simulink model "Single_track_Drift_model"  (R2024b)
settings: Solver=ode45  StartTime=0.0  StopTime=10.0  RelTol=1e-3
settings Model: Creator=fanny  LastModifiedBy=fanny

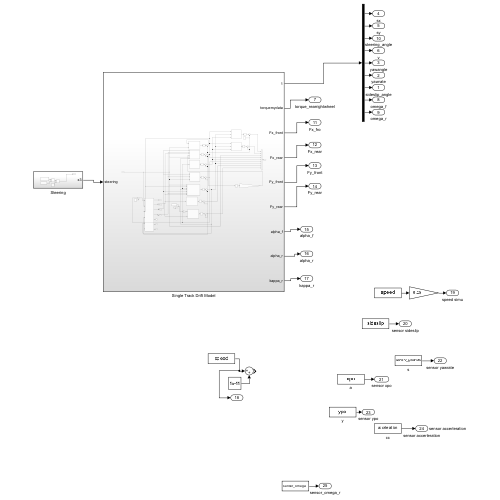
[thumbnail: Simulink's stored preview of the top-level diagram]
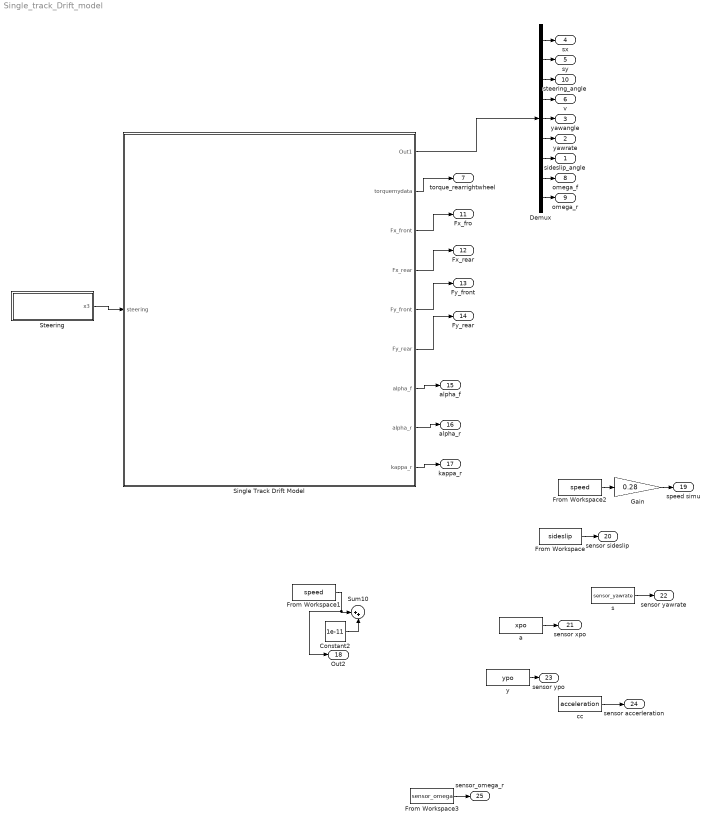
== system Single_track_Drift_model ==
  Constant2 : Constant  Value=1e-11
  Demux : Demux  Outputs=9
  From Workspace : FromWorkspace  VariableName=sideslip
  From Workspace1 : FromWorkspace  VariableName=speed
  From Workspace2 : FromWorkspace  VariableName=speed
  From Workspace3 : FromWorkspace  VariableName=sensor_omega
  Gain : Gain  Gain=0.28
  Single Track Drift Model : Subsystem
  Steering : Subsystem
  Sum10 : Sum  Inputs=|++
  a : FromWorkspace  VariableName=xpo
  cc : FromWorkspace  VariableName=acceleration
  s : FromWorkspace  VariableName=sensor_yawrate
  y : FromWorkspace  VariableName=ypo
  sideslip_angle : Outport
  yawrate : Outport  Port=2
  yawangle : Outport  Port=3
  sx : Outport  Port=4
  sy : Outport  Port=5
  v : Outport  Port=6
  torque_rearrightwheel : Outport  Port=7
  omega_f : Outport  Port=8
  omega_r : Outport  Port=9
  steering_angle : Outport  Port=10
  Fx_fro : Outport  Port=11
  Fx_rear : Outport  Port=12
  Fy_front : Outport  Port=13
  Fy_rear : Outport  Port=14
  alpha_f : Outport  Port=15
  alpha_r : Outport  Port=16
  kappa_r : Outport  Port=17
  Out2 : Outport  Port=18
  speed simu : Outport  Port=19
  sensor sideslip : Outport  Port=20
  sensor xpo : Outport  Port=21
  sensor yawrate : Outport  Port=22
  sensor ypo : Outport  Port=23
  sensor accerleration : Outport  Port=24  SignalName=sensor accerleration
  sensor_omega_r : Outport  Port=25
  wires:
  Single Track Drift Model/1(Out1) -> Demux/1
  Demux/7 -> sideslip_angle/1
  Demux/6 -> yawrate/1
  Demux/5 -> yawangle/1
  Demux/1 -> sx/1
  Demux/2 -> sy/1
  Demux/4 -> v/1
  Steering/1(x3) -> Single Track Drift Model/1(steering)
  Single Track Drift Model/2(torquemydata) -> torque_rearrightwheel/1
  Demux/8 -> omega_f/1
  Demux/9 -> omega_r/1
  Demux/3 -> steering_angle/1
  Single Track Drift Model/3(Fx_front) -> Fx_fro/1
  Single Track Drift Model/4(Fx_rear) -> Fx_rear/1
  Single Track Drift Model/5(Fy_front) -> Fy_front/1
  Single Track Drift Model/6(Fy_rear) -> Fy_rear/1
  Single Track Drift Model/7(alpha_f) -> alpha_f/1
  Single Track Drift Model/8(alpha_r) -> alpha_r/1
  Single Track Drift Model/9(kappa_r) -> kappa_r/1
  From Workspace1/1 -> Out2/1, Sum10/1
  Constant2/1 -> Sum10/2
  From Workspace2/1 -> Gain/1
  Gain/1 -> speed simu/1
  From Workspace/1 -> sensor sideslip/1
  s/1 -> sensor yawrate/1
  a/1 -> sensor xpo/1
  y/1 -> sensor ypo/1
  cc/1 -> sensor accerleration/1
  From Workspace3/1 -> sensor_omega_r/1

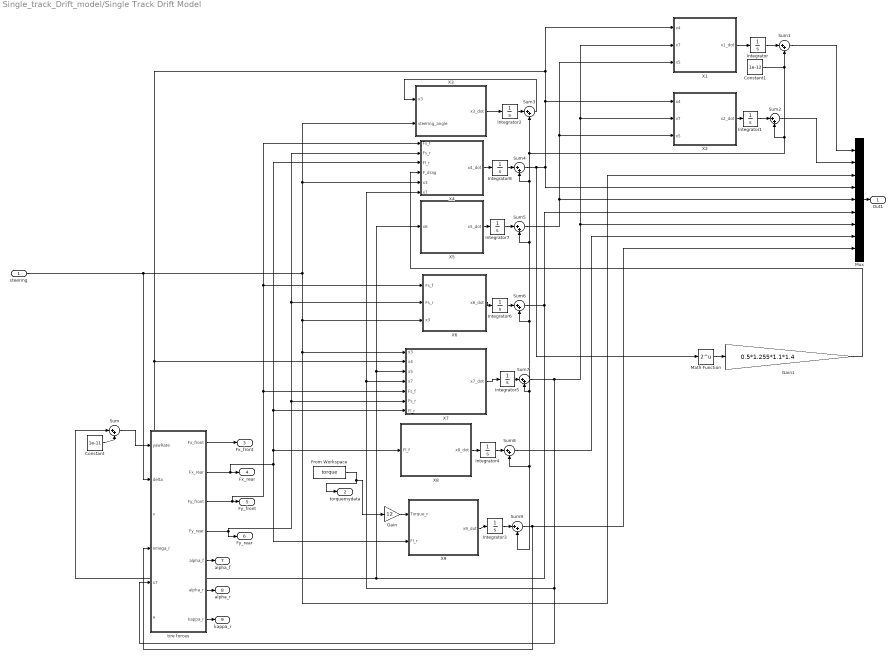
== system Single_track_Drift_model/Single Track Drift Model ==
  steering : Inport
  Constant : Constant  Value=1e-11
  Constant1 : Constant  Value=1e-12
  From Workspace : FromWorkspace  VariableName=torque
  Gain : Gain  Gain=12
  Gain1 : Gain  Gain=0.5*1.255*1.1*1.4
  Integrator{,1..2,4..7} (7 alike) : Integrator
  Integrator3 : Integrator  InitialCondition=0.1/0.26
  Integrator8 : Integrator  InitialCondition=0.1
  Math Function : Math  Operator=2^u
  Mux : Mux  Inputs=9
  Sum{,1..9} (10 alike) : Sum  Inputs=|++
  X1 : MATLAB Function  TreatAsAtomicUnit=on
  X2 : MATLAB Function  TreatAsAtomicUnit=on
  X3 : MATLAB Function  TreatAsAtomicUnit=on
  X4 : MATLAB Function  TreatAsAtomicUnit=on
  X5 : MATLAB Function  TreatAsAtomicUnit=on
  X6 : MATLAB Function  TreatAsAtomicUnit=on
  X7 : MATLAB Function  TreatAsAtomicUnit=on
  X8 : MATLAB Function  TreatAsAtomicUnit=on
  X9 : MATLAB Function  TreatAsAtomicUnit=on
  tire forces : MATLAB Function  TreatAsAtomicUnit=on
  Out1 : Outport
  torquemydata : Outport  Port=2
  Fx_front : Outport  Port=3
  Fx_rear : Outport  Port=4
  Fy_front : Outport  Port=5
  Fy_rear : Outport  Port=6
  alpha_f : Outport  Port=7
  alpha_r : Outport  Port=8
  kappa_r : Outport  Port=9
  wires:
  X1/1(x1_dot) -> Integrator/1
  X2/1(x2_dot) -> Integrator1/1
  X3/1(x3_dot) -> Integrator2/1
  X4/1(x4_dot) -> Integrator8/1
  X6/1(x6_dot) -> Integrator6/1
  X7/1(x7_dot) -> Integrator5/1
  X8/1(x8_dot) -> Integrator4/1
  X9/1(x9_dot) -> Integrator3/1
  Sum4/1 -> Math Function/1, tire forces/3(v), X7/2(x4), X1/1(x4), X2/1(x4), Mux/4
  Sum7/1 -> tire forces/5(x7), X4/6(x7), X7/4(x7), X1/2(x7), X2/2(x7), Mux/7
  Sum5/1 -> X1/3(x5), X2/3(x5), Mux/5
  Sum3/1 -> X3/1(x3)
  Sum6/1 -> X5/1(x6), X7/3(x5), Sum/1, Mux/6
  steering/1 -> X3/2(steering_angle), X4/5(x3), X6/3(x3), Mux/3, X7/1(x3), tire forces/2(delta)
  Mux/1 -> Out1/1
  Sum1/1 -> Mux/1
  Sum2/1 -> Mux/2
  Sum8/1 -> Mux/8
  Sum9/1 -> tire forces/4(omega_r), Mux/9
  tire forces/3(Fy_front) -> X4/1(Fs_f), X6/1(Fs_f), X7/5(Fs_f), Fy_front/1
  tire forces/4(Fy_rear) -> Fy_rear/1, X4/2(Fs_r), X6/2(Fs_r), X7/6(Fs_r)
  tire forces/1(Fx_front) -> Fx_front/1
  tire forces/2(Fx_rear) -> X9/2(Fl_r), X4/3(Fl_r), X7/7(Fl_r), X8/1(Fl_f), Fx_rear/1
  Sum/1 -> tire forces/1(yawRate)
  Constant/1 -> Sum/2
  Integrator/1 -> Sum1/1
  Integrator1/1 -> Sum2/1
  Constant1/1 -> Sum3/2, Sum4/2, Sum5/2, Sum6/2, Sum8/2, Sum9/2, Sum7/2, Sum2/2, Sum1/2
  Integrator2/1 -> Sum3/1
  Integrator8/1 -> Sum4/1
  Integrator7/1 -> Sum5/1
  Integrator6/1 -> Sum6/1
  Integrator5/1 -> Sum7/1
  Integrator4/1 -> Sum8/1
  Integrator3/1 -> Sum9/1
  From Workspace/1 -> Gain/1, torquemydata/1
  X5/1(x5_dot) -> Integrator7/1
  tire forces/5(alpha_f) -> alpha_f/1
  tire forces/6(alpha_r) -> alpha_r/1
  tire forces/7(kappa_r) -> kappa_r/1
  Gain/1 -> X9/1(Torque_r)
  Math Function/1 -> Gain1/1
  Gain1/1 -> X4/4(F_drag)

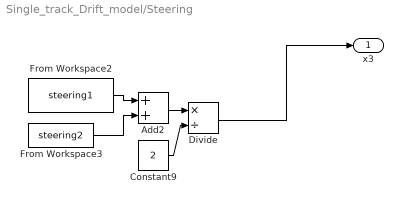
== system Single_track_Drift_model/Steering ==
  Add2 : Sum
  Constant9 : Constant  Value=2
  Divide : Product  Inputs=*/
  From Workspace2 : FromWorkspace  VariableName=steering1
  From Workspace3 : FromWorkspace  VariableName=steering2
  x3 : Outport
  wires:
  From Workspace3/1 -> Add2/2
  Constant9/1 -> Divide/2
  Divide/1 -> x3/1
  From Workspace2/1 -> Add2/1
  Add2/1 -> Divide/1

== matlab function Single_track_Drift_model/Single Track Drift Model/X9 ==
  data: x9_dot output; Torque_r input; Fl_r input
function x9_dot = compute_omega_r_dot(Torque_r, Fl_r)
% Eingaben:
% Torque_r: Antriebsmoment an der Hinterachse
% Fl_r: Längskraft an der Hinterachse
% Iy_w: Trägheitsmoment des Rades
%
% Ausgabe:
% x9_dot: Ableitung von x9
Rw = 0.26;
Iw = 10*Rw^2;

% Zustandsgleichung für x9
x9_dot = (1 / Iw) * ( -Torque_r + (Fl_r/2 * Rw));
end

== matlab function Single_track_Drift_model/Single Track Drift Model/tire forces ==
  data: Fx_front output; Fx_rear output; yawRate input; delta input; Fy_front output; Fy_rear output; v input; omega_r input; x7 input; a input; alpha_f output; alpha_r output; kappa_r output
function [Fx_front, Fx_rear, Fy_front, Fy_rear, alpha_f, alpha_r, kappa_r] = calculateTireForces(yawRate, delta, v, omega_r, x7, a)
    % Berechnet die Reifenkräfte basierend auf Fahrzeugparametern und dynamischen Werten
    Fz = 2900 / 4;
    gamma = 0.0;
    Rw = 0.26035; % Reifenradius [m]
    vx = cos(delta)*v;
    L = 1.570; %[m] wheel base
    lf = 0.874; %[m] distance from center of mass to front axle
    lr = L-lf; %[m] distance from center of mass to rear axle

    % Longitudinal parameters
    pCx1 = 1.839;
    pDx1 = 1.1387;
    pKx1 = 18.886;
    pEx1 = 0.62727;
    pHx1 = -0.00033912;
    pVx1 = -4.638e-006;

    % Lateral parameters
    pCy1 = 1.322298;
    pDy1 = 1.216919;
    pKy1 = -19.79695;
    pEy1 = -0.637732;
    pHy1 = 0.00114529;
    pVy1 = 0.0375659;

    % Calculate slip angle alpha for both axles
    alpha_f = atan((v * sin(x7) + yawRate * lf) / v * cos(x7)) - delta;
    alpha_r = atan((v * sin(x7) - yawRate * lr) / max(v * cos(x7), 1e-7));

    % Calculate longitudinal slip kappa for both axles

    kappa_r = ((vx - Rw * omega_r) / vx); %original Pacejka 2002 paper
    % Calculate longitudinal forces (Fx)
    SHx = pHx1;
    SVx = Fz * pVx1;
    
    Fx_r = calculateFx(kappa_r, SHx, SVx, Fz, pDx1, pCx1, pEx1, pKx1);

    % Calculate lateral forces (Fy)
    SHy = pHy1 + gamma * 0.044112; % pHy3 from the VI-Grade tire file
    SVy = Fz * (pVy1 + gamma * -0.3293);

    Fy_f = calculateFy(alpha_f, SHy, SVy, Fz, pDy1, pCy1, pEy1, pKy1, gamma);
    Fy_r = calculateFy(alpha_r, SHy, SVy, Fz, pDy1, pCy1, pEy1, pKy1, gamma);

    % Combine forces for front and rear
    Fx_front = 0;
    Fx_rear = 2 * Fx_r;
    Fy_front = 2 * Fy_f - 21.6;
    Fy_rear = 2 * Fy_r - 21.6;

end

function Fx = calculateFx(kappa, SHx, SVx, Fz, pDx1, pCx1, pEx1, pKx1)
    kappa_x = kappa + SHx;
    mu_x = pDx1;
    Dx = mu_x * Fz;
    Cx = pCx1;
    Kx = Fz * pKx1;
    Bx = Kx / (Cx * Dx);
    Fx = Dx * sin(Cx * atan(Bx * kappa_x - pEx1 * (Bx * kappa_x - atan(Bx * kappa_x)))) + SVx;
end

function Fy = calculateFy(alpha, SHy, SVy, Fz, pDy1, pCy1, pEy1, pKy1, gamma)
    alpha_y = alpha + SHy;
    mu_y = pDy1 * (1 - (-2.8821) * gamma^2);
    Dy = mu_y * Fz;
    Cy = pCy1;
    Ky = Fz * pKy1;
    By = Ky / (Cy * Dy);
    Fy = Dy * sin(Cy * atan(By * alpha_y - pEy1 * (By * alpha_y - atan(By * alpha_y)))) + SVy;
end

== matlab function Single_track_Drift_model/Single Track Drift Model/X2 ==
  data: x4 input; x2_dot output; x7 input; x5 input
function x2_dot = compute_sy_dot(x4, x7, x5)
% Eingaben:
% x4: Zustand x4
% x7: Zustand x7
% x5: Zustand x5
%
% Ausgabe:
% x2_dot: Ableitung von x2

% Zustandsgleichung für x2
x2_dot = 18/3.6 * sin(x7 + x5);
end

== matlab function Single_track_Drift_model/Single Track Drift Model/X1 ==
  data: x4 input; x1_dot output; x7 input; x5 input
function x1_dot = compute_sx_dot(x4, x7, x5)
% Eingaben:
% x4, x7, x5: Zustände des Systems
%
% Ausgabe:
% x1_dot: Ableitung von x1

% Zustandsgleichung
x1_dot = 18/3.6 * cos(x7 + x5);
end

== matlab function Single_track_Drift_model/Single Track Drift Model/X3 ==
  data: x3 input; x3_dot output; steering_angle input
function x3_dot = compute_steering_angle_dot(x3, steering_angle)
% Eingaben:
% x3: Zustand x3
% u1: Eingangsgröße (z.B. Lenkwinkel)
%
% Ausgabe:
% x3_dot: Ableitung von x3

% Beispiel für f_steer: Die genaue Definition musst du anpassen
x3_dot = f_steer(x3, steering_angle);
end

function f = f_steer(x3, steering_angle)
% Hilfsfunktion für f_steer
% Definiere hier die Funktion f_steer abhängig von x3 und u1
f = steering_angle - x3; % Beispiel: Differenz zwischen Eingabe und Zustand
end

== matlab function Single_track_Drift_model/Single Track Drift Model/X4 ==
  data: Fs_f input; Fs_r input; Fl_r input; F_drag input; x3 input; x4_dot output; x7 input
function x4_dot = compute_velocity_dot(Fs_f, Fs_r, Fl_r, F_drag, x3, x7)
% Eingaben:
% Fs_f: Seitliche Kraft vorne
% Fs_r: Seitliche Kraft hinten
% Fl_r: Längskraft hinten
% Fl_f: Längskraft vorne
% x3: Zustand steering angle
% x7: Zustand sideslip angle
%
% Ausgabe:
% x4_dot: Ableitung von velocity

m = 290; % in kg

% Zustandsgleichung für x4
v = (1/m) * (-Fs_f * sin(x3 - x7) + Fs_r * sin(x7) + Fl_r * cos(x7) - F_drag);

x4_dot = v;
end

== matlab function Single_track_Drift_model/Single Track Drift Model/X5 ==
  data: x6 input; x5_dot output
function x5_dot = compute_yaw_angle_dot(x6)
% Eingabe:
% x6: Zustand x6
%
% Ausgabe:
% x5_dot: Ableitung von x5

% Zustandsgleichung für x5
x5_dot = x6;
end

== matlab function Single_track_Drift_model/Single Track Drift Model/X6 ==
  data: Fs_f input; Fs_r input; x3 input; x6_dot output
function x6_dot = compute_yaw_rate_dot(Fs_f, Fs_r, x3)
% Eingaben:
% Fs_f: Seitliche Kraft vorne
% Fs_r: Seitliche Kraft hinten
% Fl_f: Längskraft vorne
% x3: Zustand steering angle
% x4: Zustand velocity
%
% Ausgabe:
% x6_dot: Ableitung von x6
Iz = 124.403600; %[kg*m^2] yaw polar inertia 
L = 1.570; %[m] wheel base
l_f =0.874; %[m] distance from center of mass to front axle
l_r = L-l_f; %[m] distance from center of mass to rear axle

% Zustandsgleichung für x6
x6_dot = (1 / Iz) * (Fs_f * cos(x3) * l_f - Fs_r * l_r);
end

== matlab function Single_track_Drift_model/Single Track Drift Model/X7 ==
  data: x3 input; x4 input; x5 input; x7 input; Fs_f input; Fs_r input; Fl_r input; x7_dot output
function x7_dot = compute_sideslip_angle_dot(x3, x4, x5, x7, Fs_f, Fs_r, Fl_r)
% Eingaben:
% x5: yawrate
% x4: velocity
% Fs_f: Seitliche Kraft vorne
% Fs_r: Seitliche Kraft hinten
% Fl_r: Längskraft hinten
% Fl_f: Längskraft vorne
% x3: steering angle
% x7: sideslip
%
% Ausgabe:
% x7_dot: Ableitung von x7
m = 290;
% Zustandsgleichung für x7
forces = (Fs_f * cos(x3 - x7) + Fs_r * cos(x7) - Fl_r * sin(x7));
x7_dot = -x5 + (1 / (m * x4)) * forces;
end

== matlab function Single_track_Drift_model/Single Track Drift Model/X8 ==
  data: x8_dot output; Fl_f input
function x8_dot = compute_omega_f_dot(Fl_f)
% Eingaben:
% Fl_f: Längskraft an der Vorderachse
% Iy_w: Trägheitsmoment des Rades
%
% Ausgabe:
% x8_dot: Ableitung von x8
Rw = 0.26;
Iw = 7*Rw^2;
% Zustandsgleichung für x8

x8_dot = 0;
end
